simulink model "mathematical_modelling_of_boost_Converter"  (R2019a)
settings: Solver=VariableStepAuto  StartTime=0.0  StopTime=0.1  RelTol=1e-3
settings Model: Creator=Deepak  LastModifiedBy=Deepak

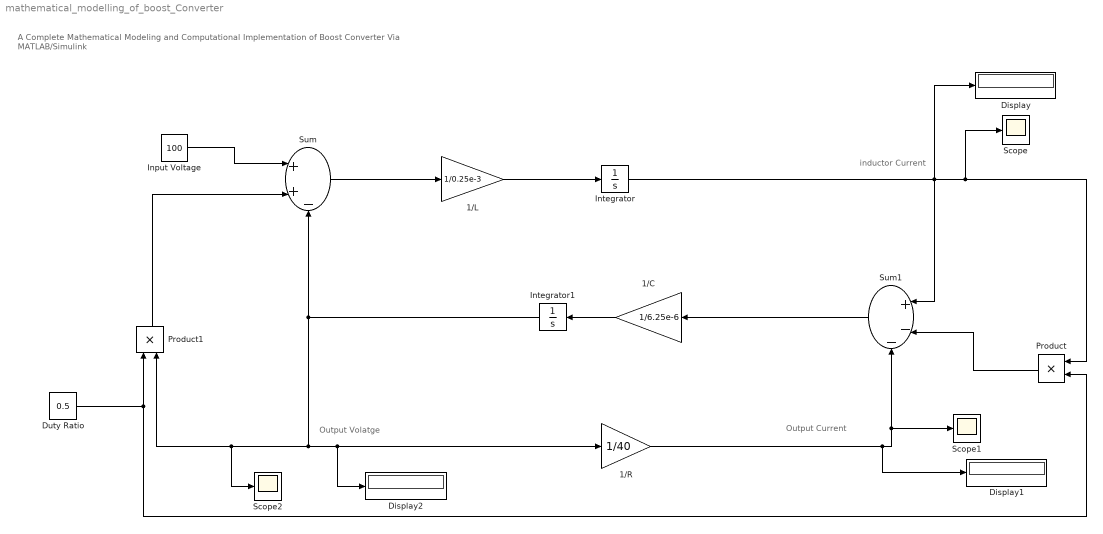
== system mathematical_modelling_of_boost_Converter ==
  note: Output Volatge
  note: Output Current
  note: inductor Current
  note: A Complete Mathematical Modeling and Computational Implementation of Boost Converter Via MATLAB/Simulink
  1/C : Gain  Gain=1/6.25e-6
  1/L : Gain  Gain=1/0.25e-3
  1/R : Gain  Gain=1/40
  Display : Display
  Display1 : Display
  Display2 : Display
  Duty Ratio : Constant  Value=0.5
  Input Voltage : Constant  Value=100
  Integrator : Integrator
  Integrator1 : Integrator
  Product : Product
  Product1 : Product
  Scope : Scope
  Scope1 : Scope
  Scope2 : Scope
  Sum : Sum  Inputs=|++-
  Sum1 : Sum  Inputs=|+--
  wires:
  Input Voltage/1 -> Sum/1
  Sum/1 -> 1/L/1
  1/L/1 -> Integrator/1
  Integrator/1 -> Display/1, Scope/1, Product/1, Sum1/1
  Sum1/1 -> 1/C/1
  1/C/1 -> Integrator1/1
  Integrator1/1 -> Display2/1, 1/R/1, Scope2/1, Product1/2, Sum/3
  1/R/1 -> Display1/1, Scope1/1, Sum1/3
  Product/1 -> Sum1/2
  Product1/1 -> Sum/2
  Duty Ratio/1 -> Product/2, Product1/1
